simulink model "sim_aut_dual_scen"  (R2025b)
settings: Solver=ode45  StartTime=0.0  StopTime=Tfin  FixedStep=1e-3  MaxStep=1e-2  MinStep=1e-3  RelTol=5e-3
values from neighbouring files (symbols this model uses):
  bp = [-1.25 -1.19897959184 -1.14795918367 -1.09693877551 -1.04591836735 -0.994897959184 -0.94387755102 -0.892857142857 -0.841836734694 -0.790816326531 -0.739795918367 -0.688775510204 ... (50 elements, 1x50)]    [tire_model.mat]
  C1 = 2.7e4    (= 27000)    [main.m]    (also in model.m)
  C2 = 2e4    (= 20000)    [main.m]    (also in model.m)
  Jz = 4000    [main.m]    (also in model.m)
  K = nmpc_design_st2(par,2)    [main.m]
  l1 = 1.2    [main.m]    (also in model.m)
  l2 = 1.6    [main.m]    (also in model.m)
  m = 1575    [main.m]    (also in model.m)
  Np = round(vx_ref*K.Tp/mean(ds))    [main.m]
  pacf = [2550.90487699 2674.70463742 2810.77279096 2960.97362657 3127.55760929 3313.26346728 3521.4532226 3756.29269015 4022.99538347 4328.15571957 4680.20907939 5090.07319782 ... (50 elements, 1x50)]    [tire_model.mat]
  pacr = [2550.90487699 2674.70463742 2810.77279096 2960.97362657 3127.55760929 3313.26346728 3521.4532226 3756.29269015 4022.99538347 4328.15571957 4680.20907939 5090.07319782 ... (50 elements, 1x50)]    [tire_model.mat]
  psi = x(3)    [model.m]
  psir = [atan2(diff(Yr),diff(Xr));0]    [main.m]
  refPoses = [Xr,Yr,psir]    [main.m]
  Ts = 0.05    [main.m]
  ze0 = [X0;Y0;psi0;vx0;vy0;wpsi0]    [main.m]
undefined symbols (not defined in the file or in its folder): aMode, plot_ref, x_o
libraries: autolibsharedcommon x11, autolibshared x5, autolibpowerinfoutils x2, autolibutils x2, sharedtransform x2, simulink x1, drivingscenarioandsensors x1
(part 2 of 4)

== system sim_aut_dual_scen/vehicle/dual-track/Vehicle Body 3DOF Dual Track/friction/mu ext dual ==
  mu_in : Inport  PortDimensions=[2,2]
  Signal Specification1 : SignalSpecification  Unit=1
  Unit Conversion2 : UnitConversion
  mu_out : Outport  PortDimensions=[2,2]  VectorParamsAs1DForOutWhenUnconnected=off
  wires:
  Signal Specification1/1 -> mu_out/1
  mu_in/1 -> Unit Conversion2/1
  Unit Conversion2/1 -> Signal Specification1/1

== system sim_aut_dual_scen/vehicle/dual-track/Vehicle Body 3DOF Dual Track/friction/mu int ==
  Constant : Constant  Value=mu
  Vector Concatenate1 : Concatenate
  mu_out : Outport  VectorParamsAs1DForOutWhenUnconnected=off
  wires:
  Constant/1 -> Vector Concatenate1/1, Vector Concatenate1/2
  Vector Concatenate1/1 -> mu_out/1

== system sim_aut_dual_scen/vehicle/dual-track/Vehicle Body 3DOF Dual Track/friction/mu int dual ==
  Constant : Constant  Value=mu
  Vector Concatenate2 : Concatenate  Mode=Multidimensional array  ConcatenateDimension=2
  Vector Concatenate3 : Concatenate  Mode=Multidimensional array  ConcatenateDimension=2
  Vector Concatenate4 : Concatenate  Mode=Multidimensional array
  mu_out : Outport  VectorParamsAs1DForOutWhenUnconnected=off
  wires:
  Vector Concatenate2/1 -> Vector Concatenate4/1
  Vector Concatenate3/1 -> Vector Concatenate4/2
  Vector Concatenate4/1 -> mu_out/1
  Constant/1 -> Vector Concatenate3/2, Vector Concatenate3/1, Vector Concatenate2/2, Vector Concatenate2/1

== system sim_aut_dual_scen/vehicle/dual-track/Vehicle Body 3DOF Dual Track/front forces/ext ==
  F_in : Inport  PortDimensions=2
  Signal Specification1 : SignalSpecification  Unit=N
  Unit Conversion3 : UnitConversion
  F_out : Outport  Unit=N  VectorParamsAs1DForOutWhenUnconnected=off
  wires:
  Signal Specification1/1 -> F_out/1
  F_in/1 -> Unit Conversion3/1
  Unit Conversion3/1 -> Signal Specification1/1

== system sim_aut_dual_scen/vehicle/dual-track/Vehicle Body 3DOF Dual Track/front forces/ext dual ==
  F_in : Inport  PortDimensions=[2,2]
  Signal Specification1 : SignalSpecification  Unit=N
  Unit Conversion3 : UnitConversion
  F_out : Outport  Unit=N  PortDimensions=[2,2]  VectorParamsAs1DForOutWhenUnconnected=off
  wires:
  Signal Specification1/1 -> F_out/1
  F_in/1 -> Unit Conversion3/1
  Unit Conversion3/1 -> Signal Specification1/1

== system sim_aut_dual_scen/vehicle/dual-track/Vehicle Body 3DOF Dual Track/front forces/ext long ==
  F_in : Inport
  Ground1 : Ground
  Signal Specification : SignalSpecification  Unit=N
  Signal Specification1 : SignalSpecification  Unit=N
  Unit Conversion1 : UnitConversion
  Vector Concatenate1 : Concatenate
  F_out : Outport  Unit=N  VectorParamsAs1DForOutWhenUnconnected=off
  wires:
  Signal Specification/1 -> Vector Concatenate1/2
  F_in/1 -> Unit Conversion1/1
  Vector Concatenate1/1 -> F_out/1
  Ground1/1 -> Signal Specification/1
  Unit Conversion1/1 -> Signal Specification1/1
  Signal Specification1/1 -> Vector Concatenate1/1

== system sim_aut_dual_scen/vehicle/dual-track/Vehicle Body 3DOF Dual Track/front forces/ext long dual ==
  F_in : Inport
  Demux : Demux  Outputs=2
  Ground : Ground
  Signal Specification5 : SignalSpecification  Unit=N
  Unit Conversion2 : UnitConversion  OutputType=Inherit: Inherit via back propagation
  Vector Concatenate1 : Concatenate  Mode=Multidimensional array  ConcatenateDimension=2
  Vector Concatenate2 : Concatenate  Mode=Multidimensional array  ConcatenateDimension=2
  Vector Concatenate3 : Concatenate  Mode=Multidimensional array
  F_out : Outport  Unit=N  VectorParamsAs1DForOutWhenUnconnected=off
  wires:
  Ground/1 -> Vector Concatenate2/2, Vector Concatenate1/2
  Vector Concatenate3/1 -> F_out/1
  Vector Concatenate1/1 -> Vector Concatenate3/1
  Vector Concatenate2/1 -> Vector Concatenate3/2
  Demux/1 -> Vector Concatenate1/1
  Demux/2 -> Vector Concatenate2/1
  Unit Conversion2/1 -> Signal Specification5/1
  Signal Specification5/1 -> Demux/1
  F_in/1 -> Unit Conversion2/1

== system sim_aut_dual_scen/vehicle/dual-track/Vehicle Body 3DOF Dual Track/front forces/int ==
  Ground : Ground
  Vector Concatenate1 : Concatenate
  F_out : Outport  VectorParamsAs1DForOutWhenUnconnected=off
  wires:
  Ground/1 -> Vector Concatenate1/2, Vector Concatenate1/1
  Vector Concatenate1/1 -> F_out/1

== system sim_aut_dual_scen/vehicle/dual-track/Vehicle Body 3DOF Dual Track/front forces/int dual ==
  Ground : Ground
  Vector Concatenate2 : Concatenate  Mode=Multidimensional array  ConcatenateDimension=2
  Vector Concatenate3 : Concatenate  Mode=Multidimensional array  ConcatenateDimension=2
  Vector Concatenate4 : Concatenate  Mode=Multidimensional array
  F_out : Outport  VectorParamsAs1DForOutWhenUnconnected=off
  wires:
  Vector Concatenate2/1 -> Vector Concatenate4/1
  Vector Concatenate3/1 -> Vector Concatenate4/2
  Vector Concatenate4/1 -> F_out/1
  Ground/1 -> Vector Concatenate3/2, Vector Concatenate3/1, Vector Concatenate2/2, Vector Concatenate2/1

== system sim_aut_dual_scen/vehicle/dual-track/Vehicle Body 3DOF Dual Track/front steer/delta ext ==
  delta_in : Inport  Unit=rad
  Signal Specification1 : SignalSpecification  Unit=rad
  Unit Conversion1 : UnitConversion
  delta_out : Outport  VectorParamsAs1DForOutWhenUnconnected=off
  wires:
  Signal Specification1/1 -> delta_out/1
  Unit Conversion1/1 -> Signal Specification1/1
  delta_in/1 -> Unit Conversion1/1

== system sim_aut_dual_scen/vehicle/dual-track/Vehicle Body 3DOF Dual Track/front steer/delta ext dual ==
  delta_in : Inport  PortDimensions=2
  Signal Specification1 : SignalSpecification  Unit=rad
  Unit Conversion2 : UnitConversion
  delta_out : Outport  Unit=rad  PortDimensions=2  VectorParamsAs1DForOutWhenUnconnected=off
  wires:
  Signal Specification1/1 -> delta_out/1
  Unit Conversion2/1 -> Signal Specification1/1
  delta_in/1 -> Unit Conversion2/1

== system sim_aut_dual_scen/vehicle/dual-track/Vehicle Body 3DOF Dual Track/front steer/delta int ==
  Ground : Ground
  delta_out : Outport  VectorParamsAs1DForOutWhenUnconnected=off
  wires:
  Ground/1 -> delta_out/1

== system sim_aut_dual_scen/vehicle/dual-track/Vehicle Body 3DOF Dual Track/front steer/delta int dual ==
  Constant : Constant  Value=0
  Vector Concatenate4 : Concatenate
  delta_out : Outport  VectorParamsAs1DForOutWhenUnconnected=off
  wires:
  Constant/1 -> Vector Concatenate4/1, Vector Concatenate4/2
  Vector Concatenate4/1 -> delta_out/1

== system sim_aut_dual_scen/vehicle/dual-track/Vehicle Body 3DOF Dual Track/hitch geometry parameters/hitch active bicycle ==
  Constant : Constant  Value=dh
  Constant1 : Constant  Value=hh
  Ground : Ground
  dh_out : Outport  VectorParamsAs1DForOutWhenUnconnected=off
  hh_out : Outport  Port=2  VectorParamsAs1DForOutWhenUnconnected=off
  hl_out : Outport  Port=3  VectorParamsAs1DForOutWhenUnconnected=off
  wires:
  Ground/1 -> hl_out/1
  Constant1/1 -> hh_out/1
  Constant/1 -> dh_out/1

== system sim_aut_dual_scen/vehicle/dual-track/Vehicle Body 3DOF Dual Track/hitch geometry parameters/hitch active dual track ==
  Constant : Constant  Value=dh
  Constant1 : Constant  Value=hh
  Constant2 : Constant  Value=hl
  dh_out : Outport  VectorParamsAs1DForOutWhenUnconnected=off
  hh_out : Outport  Port=2  VectorParamsAs1DForOutWhenUnconnected=off
  hl_out : Outport  Port=3  VectorParamsAs1DForOutWhenUnconnected=off
  wires:
  Constant2/1 -> hl_out/1
  Constant1/1 -> hh_out/1
  Constant/1 -> dh_out/1

== system sim_aut_dual_scen/vehicle/dual-track/Vehicle Body 3DOF Dual Track/hitch geometry parameters/hitch inactive ==
  Ground : Ground
  dh_out : Outport  Unit=m  PortDimensions=1  VectorParamsAs1DForOutWhenUnconnected=off
  hh_out : Outport  Port=2  Unit=m  PortDimensions=1  VectorParamsAs1DForOutWhenUnconnected=off
  hl_out : Outport  Port=3  Unit=m  PortDimensions=1  VectorParamsAs1DForOutWhenUnconnected=off
  wires:
  Ground/1 -> dh_out/1, hh_out/1, hl_out/1

== system sim_aut_dual_scen/vehicle/dual-track/Vehicle Body 3DOF Dual Track/sigma/no sigma ==
  y : Inport
  Demux : Demux  Outputs=2
  Selector : Selector  InputPortWidth=4  IndexOptions=Index vector (dialog)  Indices=[1,3]  OutputSizes=1
  alpha_f : Outport  VectorParamsAs1DForOutWhenUnconnected=off
  alpha_r : Outport  Port=2  VectorParamsAs1DForOutWhenUnconnected=off
  wires:
  Demux/2 -> alpha_r/1
  Demux/1 -> alpha_f/1
  Selector/1 -> Demux/1
  y/1 -> Selector/1

== system sim_aut_dual_scen/vehicle/dual-track/Vehicle Body 3DOF Dual Track/sigma/no sigma dual ==
  y : Inport  PortDimensions=8
  Demux : Demux  Outputs=[2,2,4]
  Terminator : Terminator
  alpha_f : Outport  VectorParamsAs1DForOutWhenUnconnected=off
  alpha_r : Outport  Port=2  VectorParamsAs1DForOutWhenUnconnected=off
  wires:
  y/1 -> Demux/1
  Demux/1 -> alpha_f/1
  Demux/2 -> alpha_r/1
  Demux/3 -> Terminator/1

== system sim_aut_dual_scen/vehicle/dual-track/Vehicle Body 3DOF Dual Track/sigma/sigma ==
  y : Inport
  Constant1 : Constant  Value=sigma_f
  Constant2 : Constant  Value=sigma_r
  Demux : Demux
  relaxation front : Subsystem
  relaxation rear : Subsystem
  alpha_f : Outport  VectorParamsAs1DForOutWhenUnconnected=off
  alpha_r : Outport  Port=2  VectorParamsAs1DForOutWhenUnconnected=off
  wires:
  Demux/3 -> relaxation rear/1(alpha)
  y/1 -> Demux/1
  Constant1/1 -> relaxation front/3(sigma)
  Constant2/1 -> relaxation rear/3(sigma)
  Demux/2 -> relaxation front/2(V)
  Demux/4 -> relaxation rear/2(V)
  relaxation rear/1(alpha_sig) -> alpha_r/1
  Demux/1 -> relaxation front/1(alpha)
  relaxation front/1(alpha_sig) -> alpha_f/1

== system sim_aut_dual_scen/vehicle/dual-track/Vehicle Body 3DOF Dual Track/sigma/sigma dual ==
  y : Inport  PortDimensions=8
  Constant1 : Constant  Value=sigma_f
  Constant2 : Constant  Value=sigma_r
  Demux : Demux  Outputs=[4,4]
  Demux1 : Demux  Outputs=[2,2]
  Vector Concatenate : Concatenate  NumInputs=4
  relaxation : Subsystem
  alpha_f : Outport  VectorParamsAs1DForOutWhenUnconnected=off
  alpha_r : Outport  Port=2  VectorParamsAs1DForOutWhenUnconnected=off
  wires:
  relaxation/1(alpha_sig) -> Demux1/1
  Demux/1 -> relaxation/1(alpha)
  Demux/2 -> relaxation/2(V)
  y/1 -> Demux/1
  Constant1/1 -> Vector Concatenate/2, Vector Concatenate/1
  Constant2/1 -> Vector Concatenate/3, Vector Concatenate/4
  Vector Concatenate/1 -> relaxation/3(sigma)
  Demux1/1 -> alpha_f/1
  Demux1/2 -> alpha_r/1

== system sim_aut_dual_scen/vehicle/dual-track/Vehicle Body 3DOF Dual Track/sigma1/no sigma ==
  y : Inport
  Demux : Demux  Outputs=2
  Selector : Selector  InputPortWidth=4  IndexOptions=Index vector (dialog)  Indices=[1,3]  OutputSizes=1
  alpha_f : Outport  VectorParamsAs1DForOutWhenUnconnected=off
  alpha_r : Outport  Port=2  VectorParamsAs1DForOutWhenUnconnected=off
  wires:
  y/1 -> Selector/1
  Selector/1 -> Demux/1
  Demux/1 -> alpha_f/1
  Demux/2 -> alpha_r/1

== system sim_aut_dual_scen/vehicle/dual-track/Vehicle Body 3DOF Dual Track/sigma1/no sigma dual ==
  y : Inport  PortDimensions=8
  Demux : Demux  Outputs=[2,2,4]
  Terminator : Terminator
  alpha_f : Outport  VectorParamsAs1DForOutWhenUnconnected=off
  alpha_r : Outport  Port=2  VectorParamsAs1DForOutWhenUnconnected=off
  wires:
  Demux/3 -> Terminator/1
  Demux/2 -> alpha_r/1
  Demux/1 -> alpha_f/1
  y/1 -> Demux/1

== system sim_aut_dual_scen/vehicle/dual-track/Vehicle Body 3DOF Dual Track/sigma1/sigma ==
  y : Inport
  Constant1 : Constant  Value=sigma_f
  Constant2 : Constant  Value=sigma_r
  Demux : Demux
  relaxation front : Subsystem
  relaxation rear : Subsystem
  alpha_f : Outport  VectorParamsAs1DForOutWhenUnconnected=off
  alpha_r : Outport  Port=2  VectorParamsAs1DForOutWhenUnconnected=off
  wires:
  relaxation front/1(alpha_sig) -> alpha_f/1
  Demux/1 -> relaxation front/1(alpha)
  relaxation rear/1(alpha_sig) -> alpha_r/1
  Demux/4 -> relaxation rear/2(V)
  Demux/2 -> relaxation front/2(V)
  Constant2/1 -> relaxation rear/3(sigma)
  Constant1/1 -> relaxation front/3(sigma)
  y/1 -> Demux/1
  Demux/3 -> relaxation rear/1(alpha)

== system sim_aut_dual_scen/vehicle/dual-track/Vehicle Body 3DOF Dual Track/sigma1/sigma dual ==
  y : Inport  PortDimensions=8
  Demux : Demux  Outputs=[4,4]
  Demux1 : Demux  Outputs=[2,2]
  Terminator : Terminator
  relaxation : Subsystem
  alpha_f : Outport  VectorParamsAs1DForOutWhenUnconnected=off
  alpha_r : Outport  Port=2  VectorParamsAs1DForOutWhenUnconnected=off
  wires:
  Demux1/2 -> alpha_r/1
  Demux1/1 -> alpha_f/1
  y/1 -> Demux/1
  Demux/1 -> relaxation/1(alpha)
  relaxation/1(alpha_sig) -> Demux1/1
  Demux/2 -> Terminator/1

== system sim_aut_dual_scen/vehicle/dual-track/Vehicle Body 3DOF Dual Track/state/xdot ext ==
  xdot : Inport
  xddot_in : Inport  Port=2  PortDimensions=4
  extState : Inport  Port=3
  Integrator : Integrator  InitialConditionSource=external  InitialCondition=[x_o;ydot_o;psi;r_o;x_o;xdot_o]
  Selector : Selector  InputPortWidth=4  IndexOptions=Index vector (dialog)  Indices=[2:4]  OutputSizes=1
  Selector1 : Selector  InputPortWidth=4  IndexOptions=Index vector (dialog)  Indices=[2:4]  OutputSizes=1
  Signal Specification : SignalSpecification  Unit=m/s
  Unit Conversion6 : UnitConversion
  Vector Concatenate : Concatenate
  Vector Concatenate1 : Concatenate
  xddot_out : Outport  VectorParamsAs1DForOutWhenUnconnected=off
  wires:
  Selector1/1 -> Vector Concatenate/2
  extState/1 -> Selector1/1
  xddot_in/1 -> Integrator/1
  Vector Concatenate1/1 -> xddot_out/1
  Selector/1 -> Vector Concatenate1/2
  xdot/1 -> Unit Conversion6/1
  Vector Concatenate/1 -> Integrator/2
  Integrator/1 -> Selector/1
  Unit Conversion6/1 -> Signal Specification/1
  Signal Specification/1 -> Vector Concatenate/1, Vector Concatenate1/1

== system sim_aut_dual_scen/vehicle/dual-track/Vehicle Body 3DOF Dual Track/state/xdot int ==
  xddot_in : Inport  PortDimensions=4
  extState : Inport  Port=2
  Integrator : Integrator  InitialConditionSource=external  InitialCondition=[x_o;ydot_o;psi;r_o;x_o;xdot_o]
  xddot_out : Outport  VectorParamsAs1DForOutWhenUnconnected=off
  wires:
  extState/1 -> Integrator/2
  xddot_in/1 -> Integrator/1
  Integrator/1 -> xddot_out/1

== system sim_aut_dual_scen/vehicle/dual-track/Vehicle Body 3DOF Dual Track/wind/wind ext ==
  wind_in : Inport
  Signal Specification1 : SignalSpecification  Unit=m/s
  Unit Conversion5 : UnitConversion
  wind_out : Outport  Unit=m/s  VectorParamsAs1DForOutWhenUnconnected=off
  wires:
  Signal Specification1/1 -> wind_out/1
  wind_in/1 -> Unit Conversion5/1
  Unit Conversion5/1 -> Signal Specification1/1

== system sim_aut_dual_scen/vehicle/dual-track/Vehicle Body 3DOF Dual Track/wind/wind int ==
  Ground : Ground
  Vector Concatenate1 : Concatenate  NumInputs=3
  wind_out : Outport  Unit=m/s  VectorParamsAs1DForOutWhenUnconnected=off
  wires:
  Ground/1 -> Vector Concatenate1/1, Vector Concatenate1/2, Vector Concatenate1/3
  Vector Concatenate1/1 -> wind_out/1

== system sim_aut_dual_scen/vehicle/dual-track/Vehicle Body 3DOF Dual Track/Cy/Cy table dual/For Each Subsystem ==
  alpha_f : Inport  Partition=on  PartitionDimension=1  PartitionWidth=1  PartitionOffset=0
  alpha_r : Inport  Port=2  Partition=on  PartitionDimension=1  PartitionWidth=1  PartitionOffset=0
  Cy_f(alpha_f) : Lookup_n-D  NumberOfTableDimensions=1  BreakpointsForDimension1=alpha_f_brk  Table=Cy_f_data  ExtrapMethod=Clip  InternalRulePriority=Speed  RndMeth=Simplest
  Cy_r(alpha_r) : Lookup_n-D  NumberOfTableDimensions=1  BreakpointsForDimension1=alpha_r_brk  Table=Cy_r_data  ExtrapMethod=Clip  InternalRulePriority=Speed  RndMeth=Simplest
  For Each : ForEach  DisableCoverage=on
  Cy_f : Outport  ConcatenationDimension=1  VectorParamsAs1DForOutWhenUnconnected=off
  Cy_r : Outport  Port=2  ConcatenationDimension=1  VectorParamsAs1DForOutWhenUnconnected=off
  wires:
  Cy_r(alpha_r)/1 -> Cy_r/1
  alpha_r/1 -> Cy_r(alpha_r)/1
  Cy_f(alpha_f)/1 -> Cy_f/1
  alpha_f/1 -> Cy_f(alpha_f)/1

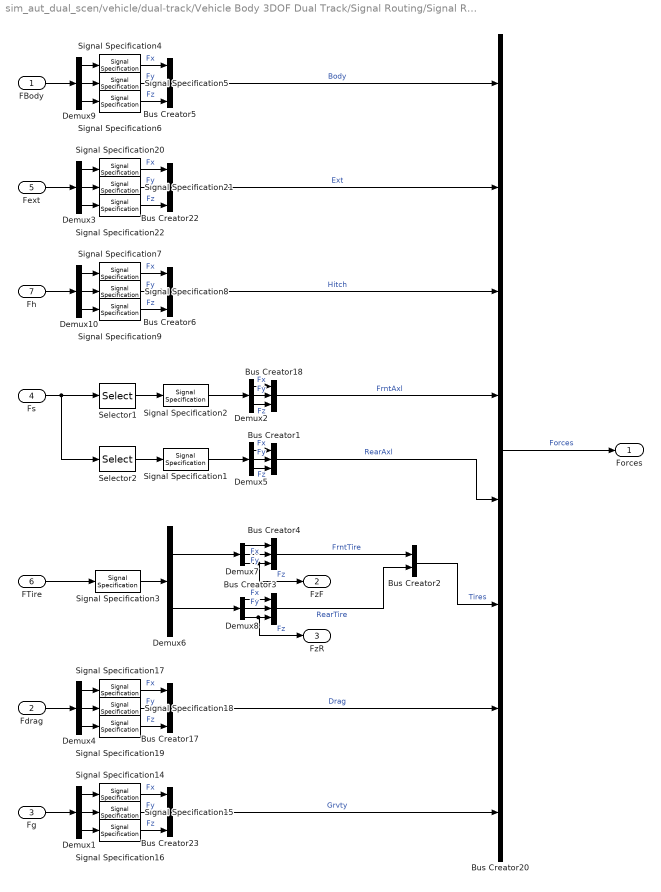
== system sim_aut_dual_scen/vehicle/dual-track/Vehicle Body 3DOF Dual Track/Signal Routing/Signal Routing/Forces 3DOF ==
  FBody : Inport
  Fdrag : Inport  Port=2
  Fg : Inport  Port=3
  Fs : Inport  Port=4  Unit=N
  Fext : Inport  Port=5
  FTire : Inport  Port=6
  Fh : Inport  Port=7  Unit=N
  Bus Creator{1,3..6,17..18,22..23} (9 alike) : BusCreator  Inputs=3
  Bus Creator2 : BusCreator  Inputs=2
  Bus Creator20 : BusCreator  Inputs=8
  Demux{1..5,7..10} (9 alike) : Demux  Outputs=3
  Demux6 : Demux  Outputs=[3,3]
  Selector1 : Selector  IndexOptions=Index vector (dialog)  Indices=[1:3]  OutputSizes=1
  Selector2 : Selector  IndexOptions=Index vector (dialog)  Indices=[4:6]  OutputSizes=1
  Signal Specification{1..9,14..22} (18 alike) : SignalSpecification  Unit=N
  Forces : Outport  VectorParamsAs1DForOutWhenUnconnected=off
  FzF : Outport  Port=2  VectorParamsAs1DForOutWhenUnconnected=off
  FzR : Outport  Port=3  VectorParamsAs1DForOutWhenUnconnected=off
  wires:
  Signal Specification8/1 -> Bus Creator6/2  "Fy"
  Fh/1 -> Demux10/1
  Signal Specification7/1 -> Bus Creator6/1  "Fx"
  Demux10/3 -> Signal Specification9/1
  Demux10/1 -> Signal Specification7/1
  Bus Creator6/1 -> Bus Creator20/3  "Hitch"
  Signal Specification9/1 -> Bus Creator6/3  "Fz"
  Demux10/2 -> Signal Specification8/1
  Signal Specification5/1 -> Bus Creator5/2  "Fy"
  Signal Specification4/1 -> Bus Creator5/1  "Fx"
  Signal Specification6/1 -> Bus Creator5/3  "Fz"
  FBody/1 -> Demux9/1
  Demux9/1 -> Signal Specification4/1
  Demux9/2 -> Signal Specification5/1
  Demux9/3 -> Signal Specification6/1
  Bus Creator5/1 -> Bus Creator20/1  "Body"
  Bus Creator17/1 -> Bus Creator20/7  "Drag"
  Bus Creator2/1 -> Bus Creator20/6  "Tires"
  Demux6/2 -> Demux8/1
  Demux6/1 -> Demux7/1
  Signal Specification3/1 -> Demux6/1
  FTire/1 -> Signal Specification3/1
  Selector2/1 -> Signal Specification1/1
  Signal Specification2/1 -> Demux2/1
  Signal Specification1/1 -> Demux5/1
  Fs/1 -> Selector2/1, Selector1/1
  Selector1/1 -> Signal Specification2/1
  Demux5/1 -> Bus Creator1/1  "Fx"
  Bus Creator4/1 -> Bus Creator2/1  "FrntTire"
  Bus Creator3/1 -> Bus Creator2/2  "RearTire"
  Demux7/1 -> Bus Creator4/1  "Fx"
  Demux7/2 -> Bus Creator4/2  "Fy"
  Demux7/3 -> Bus Creator4/3, FzF/1  "Fz"
  Demux8/3 -> Bus Creator3/3, FzR/1  "Fz"
  Demux8/2 -> Bus Creator3/2  "Fy"
  Demux8/1 -> Bus Creator3/1  "Fx"
  Demux5/2 -> Bus Creator1/2  "Fy"
  Demux5/3 -> Bus Creator1/3  "Fz"
  Demux2/3 -> Bus Creator18/3  "Fz"
  Demux2/2 -> Bus Creator18/2  "Fy"
  Demux2/1 -> Bus Creator18/1  "Fx"
  Bus Creator1/1 -> Bus Creator20/5  "RearAxl"
  Bus Creator18/1 -> Bus Creator20/4  "FrntAxl"
  Fdrag/1 -> Demux4/1
  Demux4/3 -> Signal Specification19/1
  Demux4/2 -> Signal Specification18/1
  Demux4/1 -> Signal Specification17/1
  Demux3/3 -> Signal Specification22/1
  Demux3/2 -> Signal Specification21/1
  Demux3/1 -> Signal Specification20/1
  Fext/1 -> Demux3/1
  Bus Creator22/1 -> Bus Creator20/2  "Ext"
  Signal Specification22/1 -> Bus Creator22/3  "Fz"
  Signal Specification20/1 -> Bus Creator22/1  "Fx"
  Signal Specification15/1 -> Bus Creator23/2  "Fy"
  Signal Specification21/1 -> Bus Creator22/2  "Fy"
  Signal Specification18/1 -> Bus Creator17/2  "Fy"
  Signal Specification17/1 -> Bus Creator17/1  "Fx"
  Signal Specification14/1 -> Bus Creator23/1  "Fx"
  Signal Specification19/1 -> Bus Creator17/3  "Fz"
  Signal Specification16/1 -> Bus Creator23/3  "Fz"
  Bus Creator20/1 -> Forces/1  "Forces"
  Bus Creator23/1 -> Bus Creator20/8  "Grvty"
  Demux1/2 -> Signal Specification15/1
  Demux1/3 -> Signal Specification16/1
  Fg/1 -> Demux1/1
  Demux1/1 -> Signal Specification14/1

== system sim_aut_dual_scen/vehicle/dual-track/Vehicle Body 3DOF Dual Track/Signal Routing/Signal Routing/Lateral 3DOF ==
  InertCg : Inport
  BdyFrmCg : Inport  Port=2
  Forces : Inport  Port=3
  Power : Inport  Port=4
  Moments : Inport  Port=5
  WhlAngF : Inport  Port=6  Unit=rad
  WhlAngR : Inport  Port=7  Unit=rad
  Bus Creator1 : BusCreator  Inputs=8
  Bus Creator2 : BusCreator  Inputs=5
  Bus Creator3 : BusCreator  Inputs=2
  Bus Creator4 : BusCreator  Inputs=2
  Bus Selector : BusSelector  OutputSignals=Pwr,PwrInfo
  Demux : Demux  Outputs=2
  Demux1 : Demux  Outputs=2
  Hard Point Coordinate Transform Front : autolibsharedcommon/Hard Point Coordinate Transform  R_T1=a  R_T2=0  R_T3=h  aMode=aMode
  Hard Point Coordinate Transform Geometric : Subsystem
  Hard Point Coordinate Transform Rear : autolibsharedcommon/Hard Point Coordinate Transform  R_T1=-b  R_T2=0  R_T3=h  aMode=aMode
  Hitch Coordinate Transform : Subsystem
  InertFrm : Outport  VectorParamsAs1DForOutWhenUnconnected=off
  BdyFrm : Outport  Port=2  VectorParamsAs1DForOutWhenUnconnected=off
  PwrInfo : Outport  Port=3  VectorParamsAs1DForOutWhenUnconnected=off
  wires:
  Hitch Coordinate Transform/1(Inert) -> Bus Creator2/4  "Hitch"
  Hitch Coordinate Transform/2(Body) -> Bus Creator1/6  "Hitch"
  Bus Creator2/1 -> InertFrm/1
  InertCg/1 -> Hard Point Coordinate Transform Geometric/1(InertFrmCg), Hitch Coordinate Transform/1(InertFrmCg), Hard Point Coordinate Transform Rear/1, Hard Point Coordinate Transform Front/1, Bus Creator2/1  "Cg"
  Hard Point Coordinate Transform Front/1 -> Bus Creator2/2  "FrntAxl"
  Hard Point Coordinate Transform Rear/2 -> Bus Creator1/5  "RearAxl"
  Bus Creator1/1 -> BdyFrm/1  "BdyFrm"
  Hard Point Coordinate Transform Rear/1 -> Bus Creator2/3  "RearAxl"
  Hard Point Coordinate Transform Front/2 -> Bus Creator1/4  "FrntAxl"
  Forces/1 -> Bus Creator1/2  "Forces"
  Bus Selector/1 -> Bus Creator1/7  "<Pwr>"
  Moments/1 -> Bus Creator1/3  "Moments"
  BdyFrmCg/1 -> Hard Point Coordinate Transform Front/2, Hitch Coordinate Transform/2(BodyFrmCg), Bus Creator1/1, Hard Point Coordinate Transform Geometric/2(BdyFrmCg), Hard Point Coordinate Transform Rear/2  "Cg"
  Hard Point Coordinate Transform Geometric/1(Inert) -> Bus Creator2/5  "Geom"
  Hard Point Coordinate Transform Geometric/2(Body) -> Bus Creator1/8  "Geom"
  Bus Creator3/1 -> Hard Point Coordinate Transform Front/3  "Steer"
  WhlAngF/1 -> Demux/1  "WhlAngF"
  WhlAngR/1 -> Demux1/1  "WhlAngR"
  Bus Creator4/1 -> Hard Point Coordinate Transform Rear/3  "Steer"
  Demux/2 -> Bus Creator3/2  "WhlAngFR"
  Demux1/1 -> Bus Creator4/1  "WhlAngRL"
  Demux1/2 -> Bus Creator4/2  "WhlAngRR"
  Demux/1 -> Bus Creator3/1  "WhlAngFL"
  Bus Selector/2 -> PwrInfo/1  "<PwrInfo>"
  Power/1 -> Bus Selector/1  "Pwr"

== system sim_aut_dual_scen/vehicle/dual-track/Vehicle Body 3DOF Dual Track/Signal Routing/Signal Routing/Moments ==
  MBody : Inport
  Mdrag : Inport  Port=2
  MExt : Inport  Port=3
  Mh : Inport  Port=4
  Bus Creator{1..3,24} (4 alike) : BusCreator  Inputs=3
  Bus Creator7 : BusCreator  Inputs=4
  Demux{,1..3} (4 alike) : Demux  Outputs=3
  Signal Specification{1..11,23} (12 alike) : SignalSpecification  Unit=N*m
  Moments : Outport  VectorParamsAs1DForOutWhenUnconnected=off
  wires:
  Signal Specification10/1 -> Bus Creator2/3  "Mz"
  Demux3/3 -> Signal Specification10/1
  Demux3/1 -> Signal Specification11/1
  Signal Specification11/1 -> Bus Creator2/1  "Mx"
  Mh/1 -> Demux3/1
  Demux3/2 -> Signal Specification9/1
  Signal Specification9/1 -> Bus Creator2/2  "My"
  Bus Creator2/1 -> Bus Creator7/4  "Hitch"
  Signal Specification23/1 -> Bus Creator24/1  "Mx"
  Bus Creator24/1 -> Bus Creator7/1  "Body"
  Signal Specification1/1 -> Bus Creator24/2  "My"
  Signal Specification2/1 -> Bus Creator24/3  "Mz"
  Bus Creator1/1 -> Bus Creator7/2  "Drag"
  Bus Creator7/1 -> Moments/1  "Moments"
  Demux/2 -> Signal Specification1/1
  Demux/1 -> Signal Specification23/1
  Demux/3 -> Signal Specification2/1
  MBody/1 -> Demux/1
  Mdrag/1 -> Demux1/1
  Demux1/3 -> Signal Specification4/1
  Demux1/1 -> Signal Specification5/1
  Demux1/2 -> Signal Specification3/1
  Signal Specification4/1 -> Bus Creator1/3  "Mz"
  Signal Specification3/1 -> Bus Creator1/2  "My"
  Signal Specification5/1 -> Bus Creator1/1  "Mx"
  MExt/1 -> Demux2/1
  Signal Specification7/1 -> Bus Creator3/3  "Mz"
  Signal Specification6/1 -> Bus Creator3/2  "My"
  Bus Creator3/1 -> Bus Creator7/3  "Ext"
  Signal Specification8/1 -> Bus Creator3/1  "Mx"
  Demux2/2 -> Signal Specification6/1
  Demux2/1 -> Signal Specification8/1
  Demux2/3 -> Signal Specification7/1

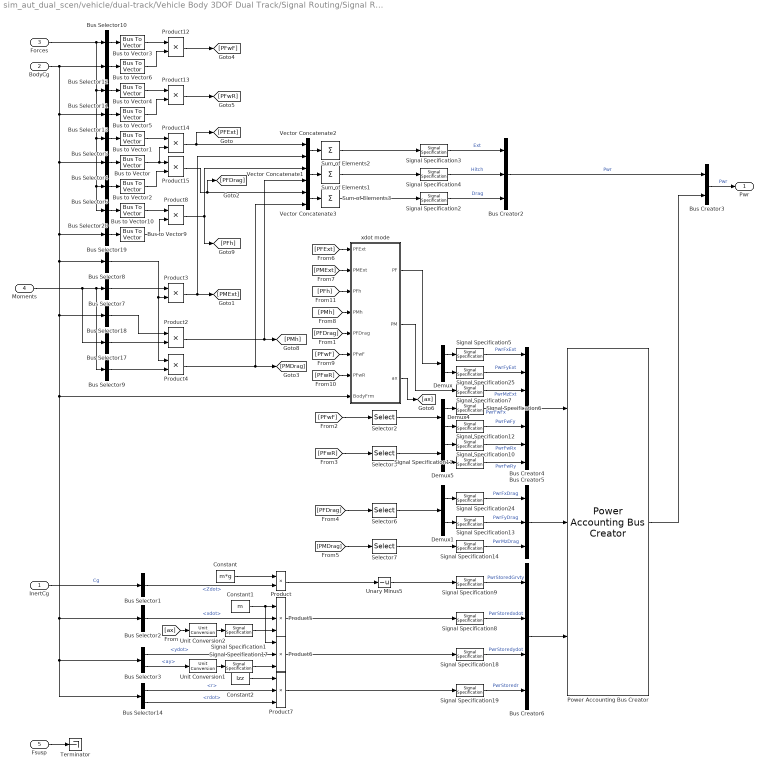
== system sim_aut_dual_scen/vehicle/dual-track/Vehicle Body 3DOF Dual Track/Signal Routing/Signal Routing/Power ==
  InertCg : Inport
  BodyCg : Inport  Port=2
  Forces : Inport  Port=3
  Moments : Inport  Port=4
  Fsusp : Inport  Port=5
  Bus Creator2 : BusCreator  Inputs=3
  Bus Creator3 : BusCreator  Inputs=2
  Bus Creator4 : BusCreator  Inputs=7
  Bus Creator5 : BusCreator  Inputs=3
  Bus Creator6 : BusCreator  Inputs=4
  Bus Selector1 : BusSelector  OutputSignals=Cg.Vel.Zdot
  Bus Selector10 : BusSelector  OutputSignals=FrntAxl.Fx,FrntAxl.Fy,FrntAxl.Fz  OutputAsBus=on
  Bus Selector11 : BusSelector  OutputSignals=RearAxl.Fx,RearAxl.Fy,RearAxl.Fz  OutputAsBus=on
  Bus Selector12 : BusSelector  OutputSignals=FrntAxl.Vel.xdot,FrntAxl.Vel.ydot,FrntAxl.Vel.zdot  OutputAsBus=on
  Bus Selector13 : BusSelector  OutputSignals=RearAxl.Vel.xdot,RearAxl.Vel.ydot,RearAxl.Vel.zdot  OutputAsBus=on
  Bus Selector14 : BusSelector  OutputSignals=Cg.AngVel.r,Cg.AngAcc.rdot
  Bus Selector17 : BusSelector  OutputSignals=Hitch.Mx,Hitch.My,Hitch.Mz  OutputAsBus=on
  Bus Selector18 : BusSelector  OutputSignals=Cg.AngVel.p,Cg.AngVel.q,Cg.AngVel.r  OutputAsBus=on
  Bus Selector19 : BusSelector  OutputSignals=Hitch.Vel.xdot,Hitch.Vel.ydot,Hitch.Vel.zdot  OutputAsBus=on
  Bus Selector2 : BusSelector  OutputSignals=Cg.Vel.xdot
  Bus Selector20 : BusSelector  OutputSignals=Hitch.Fx,Hitch.Fy,Hitch.Fz  OutputAsBus=on
  Bus Selector3 : BusSelector  OutputSignals=Cg.Vel.ydot,Cg.Acc.ay
  Bus Selector4 : BusSelector  OutputSignals=Cg.Vel.xdot,Cg.Vel.ydot,Cg.Vel.zdot  OutputAsBus=on
  Bus Selector5 : BusSelector  OutputSignals=Ext.Fx,Ext.Fy,Ext.Fz  OutputAsBus=on
  Bus Selector6 : BusSelector  OutputSignals=Drag.Fx,Drag.Fy,Drag.Fz  OutputAsBus=on
  Bus Selector7 : BusSelector  OutputSignals=Ext.Mx,Ext.My,Ext.Mz  OutputAsBus=on
  Bus Selector8 : BusSelector  OutputSignals=Cg.AngVel.p,Cg.AngVel.q,Cg.AngVel.r  OutputAsBus=on
  Bus Selector9 : BusSelector  OutputSignals=Drag.Mx,Drag.My,Drag.Mz  OutputAsBus=on
  Bus to Vector{,1..6,9..10} (9 alike) : BusToVector
  Constant : Constant  Value=m*g
  Constant1 : Constant  Value=m
  Constant2 : Constant  Value=Izz
  Demux{,1,4..5} (4 alike) : Demux  Outputs=2
  Power Accounting Bus Creator : autolibpowerinfoutils/Power Accounting Bus Creator  AssctBlkSelPopup=Parent reference block  RefBlkName='autolibshared/Vehicle Body 3DOF Single Track'  PwrTrnsfrdCheckBox=on  PwrNotTrnsfrdCheckBox=on  PwrStoredCheckBox=on  aMode=aMode
  Product{,2..4,8,12..15} (9 alike) : Product
  Product5 : Product  Inputs=3
  Product6 : Product  Inputs=3
  Product7 : Product  Inputs=3
  Selector2 : Selector  InputPortWidth=3  IndexOptions=Index vector (dialog)  Indices=[1 2]  OutputSizes=1
  Selector3 : Selector  InputPortWidth=3  IndexOptions=Index vector (dialog)  Indices=[1 2]  OutputSizes=1
  Selector6 : Selector  InputPortWidth=3  IndexOptions=Index vector (dialog)  Indices=[1 2]  OutputSizes=1
  Selector7 : Selector  InputPortWidth=3  IndexOptions=Index vector (dialog)  Indices=[3]  OutputSizes=1
  Signal Specification1 : SignalSpecification  Unit=m/s^2
  Signal Specification{2..14,18..19,24..25} (17 alike) : SignalSpecification  Unit=W
  Signal Specification17 : SignalSpecification  Unit=m/s^2
  Sum of Elements1 : Sum  Inputs=+
  Sum of Elements2 : Sum  Inputs=+
  Sum of Elements3 : Sum  Inputs=+
  Terminator : Terminator
  Unary Minus5 : UnaryMinus
  Unit Conversion1 : UnitConversion
  Unit Conversion2 : UnitConversion
  Vector Concatenate1 : Concatenate
  Vector Concatenate2 : Concatenate
  Vector Concatenate3 : Concatenate
  xdot mode : Subsystem  Variant=on  VariantControlMode=label  LabelModeActiveChoice=1
  Pwr : Outport  VectorParamsAs1DForOutWhenUnconnected=off
  wires:
  [PMh] -> xdot mode/4(PMh)
  [PFh] -> xdot mode/3(PFh)
  Vector Concatenate1/1 -> Sum of Elements1/1
  Sum of Elements1/1 -> Signal Specification4/1
  Signal Specification4/1 -> Bus Creator2/2  "Hitch"
  Bus Selector19/1 -> Bus to Vector9/1
  Bus to Vector9/1 -> Product8/2
  Bus to Vector10/1 -> Product8/1
  Bus Selector20/1 -> Bus to Vector10/1
  Product8/1 -> [PFh], Vector Concatenate1/1
  Product2/1 -> Vector Concatenate1/2, [PMh]
  BodyCg/1 -> Bus Selector4/1, Bus Selector8/1, Bus Selector18/1, xdot mode/8(BodyFrm), Bus Selector2/1, Bus Selector14/1, Bus Selector3/1, Bus Selector19/1, Bus Selector13/1, Bus Selector12/1
  Moments/1 -> Bus Selector7/1, Bus Selector9/1, Bus Selector17/1
  Bus Selector18/1 -> Product2/1
  Bus Selector17/1 -> Product2/2
  Signal Specification3/1 -> Bus Creator2/1  "Ext"
  Product15/1 -> Vector Concatenate3/1, [PFDrag]
  Bus Creator2/1 -> Bus Creator3/1  "Pwr"
  Product14/1 -> [PFExt], Vector Concatenate2/1
  Bus Selector5/1 -> Bus to Vector1/1
  Bus Selector1/1 -> Product/2  "<Zdot>"
  Product3/1 -> [PMExt], Vector Concatenate2/2
  Bus Selector11/1 -> Bus to Vector4/1
  InertCg/1 -> Bus Selector1/1  "Cg"
  Sum of Elements3/1 -> Signal Specification2/1
  Bus to Vector1/1 -> Product14/1
  Bus Selector6/1 -> Bus to Vector2/1
  Signal Specification8/1 -> Bus Creator6/2  "PwrStoredxdot"
  [PFwR] -> Selector3/1
  Demux/2 -> Signal Specification25/1
  Product13/1 -> [PFwR]
  Product7/1 -> Signal Specification19/1
  Bus Selector3/1 -> Product6/2  "<ydot>"
  Constant2/1 -> Product7/1
  Sum of Elements2/1 -> Signal Specification3/1
  Bus to Vector2/1 -> Product15/2
  Bus Selector13/1 -> Bus to Vector5/1
  Vector Concatenate2/1 -> Sum of Elements2/1
  Signal Specification19/1 -> Bus Creator6/4  "PwrStoredr"
  Bus Selector2/1 -> Product5/2  "<xdot>"
  Vector Concatenate3/1 -> Sum of Elements3/1
  Signal Specification18/1 -> Bus Creator6/3  "PwrStoredydot"
  Bus Selector14/2 -> Product7/3  "<rdot>"
  Bus Selector14/1 -> Product7/2  "<r>"
  Forces/1 -> Bus Selector6/1, Bus Selector20/1, Bus Selector5/1, Bus Selector11/1, Bus Selector10/1
  xdot mode/1(PF) -> Demux/1
  Bus Selector10/1 -> Bus to Vector3/1
  Bus to Vector6/1 -> Product12/2
  [PMDrag] -> Selector7/1
  Signal Specification14/1 -> Bus Creator5/3  "PwrMzDrag"
  [PFwF] -> Selector2/1
  Signal Specification7/1 -> Bus Creator4/3  "PwrMzExt"
  Bus Selector4/1 -> Bus to Vector/1
  Bus to Vector3/1 -> Product12/1
  Signal Specification13/1 -> Bus Creator5/2  "PwrFyDrag"
  [PFDrag] -> Selector6/1
  Selector6/1 -> Demux1/1
  Bus Selector12/1 -> Bus to Vector6/1
  Signal Specification6/1 -> Bus Creator4/4  "PwrFwFx"
  Bus Creator3/1 -> Pwr/1  "Pwr"
  Bus to Vector4/1 -> Product13/1
  Signal Specification9/1 -> Bus Creator6/1  "PwrStoredGrvty"
  Signal Specification11/1 -> Bus Creator4/7  "PwrFwRy"
  xdot mode/2(PM) -> Signal Specification7/1
  Bus Selector7/1 -> Product3/1
  Signal Specification2/1 -> Bus Creator2/3  "Drag"
  Bus Selector8/1 -> Product3/2, Product4/1
  Signal Specification10/1 -> Bus Creator4/6  "PwrFwRx"
  Signal Specification12/1 -> Bus Creator4/5  "PwrFwFy"
  Selector2/1 -> Demux4/1
  Demux5/2 -> Signal Specification11/1
  Bus Selector9/1 -> Product4/2
  Selector3/1 -> Demux5/1
  Demux4/1 -> Signal Specification6/1
  Demux1/1 -> Signal Specification24/1
  Product12/1 -> [PFwF]
  Unary Minus5/1 -> Signal Specification9/1
  Signal Specification24/1 -> Bus Creator5/1  "PwrFxDrag"
  Demux5/1 -> Signal Specification10/1
  Signal Specification5/1 -> Bus Creator4/1  "PwrFxExt"
  Bus Creator6/1 -> Power Accounting Bus Creator/3
  Bus to Vector/1 -> Product15/1, Product14/2
  Constant1/1 -> Product6/1, Product5/1
  Signal Specification25/1 -> Bus Creator4/2  "PwrFyExt"
  Product/1 -> Unary Minus5/1
  Bus Creator5/1 -> Power Accounting Bus Creator/2
  Bus to Vector5/1 -> Product13/2
  Bus Creator4/1 -> Power Accounting Bus Creator/1
  Demux/1 -> Signal Specification5/1
  Product6/1 -> Signal Specification18/1
  Constant/1 -> Product/1
  Demux4/2 -> Signal Specification12/1
  Power Accounting Bus Creator/1 -> Bus Creator3/2
  Product4/1 -> [PMDrag], Vector Concatenate3/2
  Fsusp/1 -> Terminator/1
  [PFExt] -> xdot mode/1(PFExt)
  [PMExt] -> xdot mode/2(PMExt)
  [PFDrag] -> xdot mode/5(PFDrag)
  [PFwF] -> xdot mode/6(PFwF)
  [PFwR] -> xdot mode/7(PFwR)
  Product5/1 -> Signal Specification8/1
  Signal Specification17/1 -> Product6/3
  Unit Conversion1/1 -> Signal Specification17/1
  Bus Selector3/2 -> Unit Conversion1/1  "<ay>"
  Selector7/1 -> Signal Specification14/1
  Demux1/2 -> Signal Specification13/1
  Signal Specification1/1 -> Product5/3
  Unit Conversion2/1 -> Signal Specification1/1
  xdot mode/3(ax) -> [ax]
  [ax] -> Unit Conversion2/1

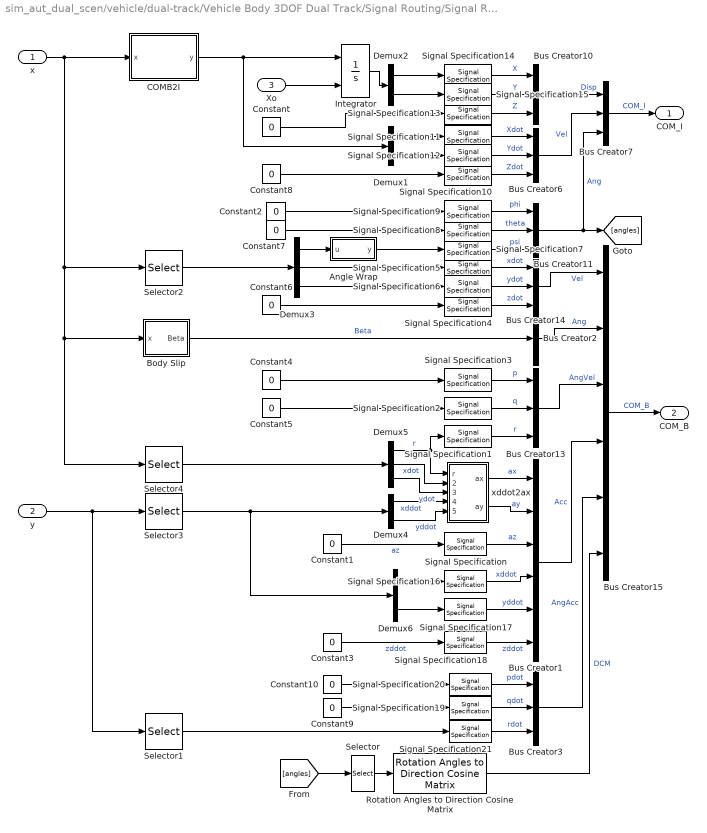
== system sim_aut_dual_scen/vehicle/dual-track/Vehicle Body 3DOF Dual Track/Signal Routing/Signal Routing/state2bus ==
  x : Inport
  y : Inport  Port=2
  Xo : Inport  Port=3
  Angle Wrap : Subsystem  Variant=on  VariantControlMode=label  VariantControl=Variant1  LabelModeActiveChoice=None
  Body Slip : Subsystem
  Bus Creator1 : BusCreator  Inputs=6
  Bus Creator{3,6..7,10..11,13..14} (7 alike) : BusCreator  Inputs=3
  Bus Creator15 : BusCreator  Inputs=6
  Bus Creator2 : BusCreator  Inputs=1
  COMB2I : MATLAB Function  TreatAsAtomicUnit=on
  Constant{,1..10} (11 alike) : Constant  Value=0
  Demux{1..2,4,6} (4 alike) : Demux  Outputs=2
  Demux3 : Demux  Outputs=3
  Demux5 : Demux  Outputs=3
  Integrator : Integrator  InitialConditionSource=external
  Rotation Angles to Direction Cosine Matrix : sharedtransform/Rotation Angles to Direction Cosine Matrix  rotationOrder=ZYX  aMode=aMode
  Selector : Selector  InputPortWidth=3  IndexOptions=Index vector (dialog)  Indices=[3 2 1]  OutputSizes=1
  Selector1 : Selector  IndexOptions=Index vector (dialog)  Indices=[3]  OutputSizes=1
  Selector2 : Selector  IndexOptions=Index vector (dialog)  Indices=[3,1,2]  OutputSizes=1
  Selector3 : Selector  IndexOptions=Index vector (dialog)  Indices=[1,2]  OutputSizes=1
  Selector4 : Selector  IndexOptions=Index vector (dialog)  Indices=[4,1,2]  OutputSizes=1
  Signal Specification : SignalSpecification  Unit=gn
  Signal Specification1 : SignalSpecification  Unit=rad/s
  Signal Specification{4..6,10..12} (6 alike) : SignalSpecification  Unit=m/s
  Signal Specification13 : SignalSpecification  Unit=m
  Signal Specification14 : SignalSpecification  Unit=m
  Signal Specification15 : SignalSpecification  Unit=m
  Signal Specification16 : SignalSpecification  Unit=m/s^2
  Signal Specification17 : SignalSpecification  Unit=m/s^2
  Signal Specification18 : SignalSpecification  Unit=m/s^2
  Signal Specification19 : SignalSpecification  Unit=rad/s^2
  Signal Specification2 : SignalSpecification  Unit=rad/s
  Signal Specification20 : SignalSpecification  Unit=rad/s^2
  Signal Specification21 : SignalSpecification  Unit=rad/s^2
  Signal Specification3 : SignalSpecification  Unit=rad/s
  Signal Specification7 : SignalSpecification  Unit=rad
  Signal Specification8 : SignalSpecification  Unit=rad
  Signal Specification9 : SignalSpecification  Unit=rad
  xddot2ax : Subsystem
  COM_I : Outport  VectorParamsAs1DForOutWhenUnconnected=off
  COM_B : Outport  Port=2  VectorParamsAs1DForOutWhenUnconnected=off
  wires:
  [angles] -> Selector/1
  Selector/1 -> Rotation Angles to Direction Cosine Matrix/1
  Rotation Angles to Direction Cosine Matrix/1 -> Bus Creator15/6  "DCM"
  Angle Wrap/1(" y") -> Signal Specification7/1
  Selector1/1 -> Signal Specification21/1
  Constant10/1 -> Signal Specification20/1
  Constant9/1 -> Signal Specification19/1
  Bus Creator3/1 -> Bus Creator15/5  "AngAcc"
  Signal Specification20/1 -> Bus Creator3/1  "pdot"
  Signal Specification19/1 -> Bus Creator3/2  "qdot"
  Signal Specification21/1 -> Bus Creator3/3  "rdot"
  Xo/1 -> Integrator/2
  Body Slip/1(Beta) -> Bus Creator2/1  "Beta"
  Bus Creator2/1 -> Bus Creator15/2  "Ang"
  Bus Creator1/1 -> Bus Creator15/4  "Acc"
  Constant8/1 -> Signal Specification10/1
  Demux6/2 -> Signal Specification17/1
  Demux6/1 -> Signal Specification16/1
  Constant1/1 -> Signal Specification/1  "az"
  Signal Specification16/1 -> Bus Creator1/4  "xddot"
  Signal Specification17/1 -> Bus Creator1/5  "yddot"
  Signal Specification18/1 -> Bus Creator1/6  "zddot"
  Constant3/1 -> Signal Specification18/1  "zddot"
  Selector3/1 -> Demux6/1, Demux4/1
  y/1 -> Selector3/1, Selector1/1
  Signal Specification/1 -> Bus Creator1/3  "az"
  Signal Specification7/1 -> Bus Creator11/3  "psi"
  COMB2I/1(y) -> Demux1/1, Integrator/1
  Integrator/1 -> Demux2/1
  Signal Specification6/1 -> Bus Creator14/2  "ydot"
  Bus Creator11/1 -> Bus Creator7/3, [angles]  "Ang"
  Signal Specification5/1 -> Bus Creator14/1  "xdot"
  Bus Creator15/1 -> COM_B/1  "COM_B"
  Signal Specification2/1 -> Bus Creator13/2  "q"
  Signal Specification12/1 -> Bus Creator6/2  "Ydot"
  Selector2/1 -> Demux3/1
  Signal Specification8/1 -> Bus Creator11/2  "theta"
  Bus Creator10/1 -> Bus Creator7/1  "Disp"
  Bus Creator6/1 -> Bus Creator7/2  "Vel"
  Bus Creator14/1 -> Bus Creator15/1  "Vel"
  Signal Specification3/1 -> Bus Creator13/1  "p"
  Bus Creator7/1 -> COM_I/1  "COM_I"
  Signal Specification9/1 -> Bus Creator11/1  "phi"
  Signal Specification14/1 -> Bus Creator10/1  "X"
  Signal Specification13/1 -> Bus Creator10/3  "Z"
  Bus Creator13/1 -> Bus Creator15/3  "AngVel"
  Signal Specification15/1 -> Bus Creator10/2  "Y"
  Signal Specification11/1 -> Bus Creator6/1  "Xdot"
  Signal Specification4/1 -> Bus Creator14/3  "zdot"
  Signal Specification10/1 -> Bus Creator6/3  "Zdot"
  x/1 -> COMB2I/1(x), Selector2/1, Body Slip/1(x), Selector4/1
  Demux5/1 -> Signal Specification1/1, xddot2ax/1(r)  "r"
  Selector4/1 -> Demux5/1
  Demux5/2 -> xddot2ax/2(xdot)  "xdot"
  Demux5/3 -> xddot2ax/3(ydot)  "ydot"
  Demux4/1 -> xddot2ax/4(xddot)  "xddot"
  Demux4/2 -> xddot2ax/5(yddot)  "yddot"
  xddot2ax/1(ax) -> Bus Creator1/1  "ax"
  xddot2ax/2(ay) -> Bus Creator1/2  "ay"
  Signal Specification1/1 -> Bus Creator13/3  "r"
  Constant5/1 -> Signal Specification2/1
  Constant4/1 -> Signal Specification3/1
  Constant6/1 -> Signal Specification4/1
  Demux3/2 -> Signal Specification5/1
  Demux3/3 -> Signal Specification6/1
  Demux3/1 -> Angle Wrap/1("u ")
  Constant7/1 -> Signal Specification8/1
  Constant2/1 -> Signal Specification9/1
  Demux1/2 -> Signal Specification12/1
  Demux1/1 -> Signal Specification11/1
  Constant/1 -> Signal Specification13/1
  Demux2/2 -> Signal Specification15/1
  Demux2/1 -> Signal Specification14/1

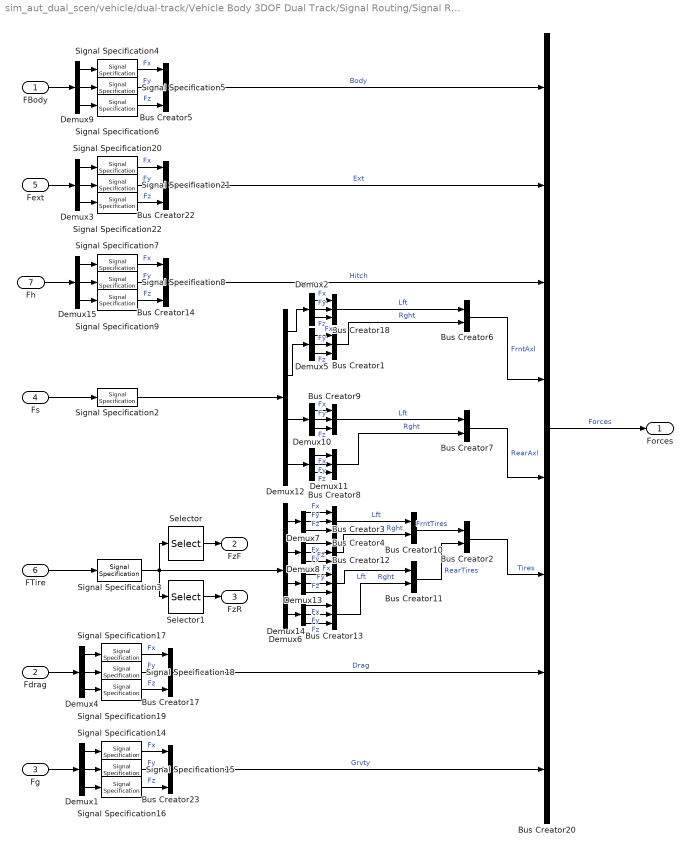
== system sim_aut_dual_scen/vehicle/dual-track/Vehicle Body 3DOF Dual Track/Signal Routing/Signal Routing Dual/Forces 3DOF ==
  FBody : Inport
  Fdrag : Inport  Port=2
  Fg : Inport  Port=3
  Fs : Inport  Port=4  Unit=N
  Fext : Inport  Port=5
  FTire : Inport  Port=6
  Fh : Inport  Port=7
  Bus Creator{1,3..5,8..9,12..14,17..18,22..23} (13 alike) : BusCreator  Inputs=3
  Bus Creator{2,6..7,10..11} (5 alike) : BusCreator  Inputs=2
  Bus Creator20 : BusCreator  Inputs=8
  Demux{1..5,7..11,13..15} (13 alike) : Demux  Outputs=3
  Demux12 : Demux  Outputs=[3,3,3,3]
  Demux6 : Demux  Outputs=[3,3,3,3]
  Selector : Selector  InputPortWidth=12  IndexOptions=Index vector (dialog)  Indices=[3,6]  OutputSizes=1
  Selector1 : Selector  InputPortWidth=12  IndexOptions=Index vector (dialog)  Indices=[9,12]  OutputSizes=1
  Signal Specification{2..9,14..22} (17 alike) : SignalSpecification  Unit=N
  Forces : Outport  VectorParamsAs1DForOutWhenUnconnected=off
  FzF : Outport  Port=2  VectorParamsAs1DForOutWhenUnconnected=off
  FzR : Outport  Port=3  VectorParamsAs1DForOutWhenUnconnected=off
  wires:
  Demux15/2 -> Signal Specification8/1
  Demux15/1 -> Signal Specification7/1
  Signal Specification9/1 -> Bus Creator14/3  "Fz"
  Signal Specification8/1 -> Bus Creator14/2  "Fy"
  Fh/1 -> Demux15/1
  Demux15/3 -> Signal Specification9/1
  Bus Creator14/1 -> Bus Creator20/3  "Hitch"
  Signal Specification7/1 -> Bus Creator14/1  "Fx"
  Selector1/1 -> FzR/1
  Selector/1 -> FzF/1
  Demux13/3 -> Bus Creator12/3  "Fz"
  Bus Creator13/1 -> Bus Creator11/2  "Rght"
  Demux14/1 -> Bus Creator13/1  "Fx"
  Demux14/2 -> Bus Creator13/2  "Fy"
  Demux14/3 -> Bus Creator13/3  "Fz"
  Demux6/4 -> Demux14/1
  Demux6/3 -> Demux13/1
  Demux13/2 -> Bus Creator12/2  "Fy"
  Demux13/1 -> Bus Creator12/1  "Fx"
  Signal Specification2/1 -> Demux12/1
  Bus Creator12/1 -> Bus Creator11/1  "Lft"
  Bus Creator3/1 -> Bus Creator10/2  "Rght"
  Bus Creator4/1 -> Bus Creator10/1  "Lft"
  Demux12/3 -> Demux10/1
  Demux12/4 -> Demux11/1
  Demux11/1 -> Bus Creator8/1  "Fx"
  Demux11/2 -> Bus Creator8/2  "Fy"
  Demux11/3 -> Bus Creator8/3  "Fz"
  Demux10/3 -> Bus Creator9/3  "Fz"
  Demux10/2 -> Bus Creator9/2  "Fy"
  Demux10/1 -> Bus Creator9/1  "Fx"
  Bus Creator9/1 -> Bus Creator7/1  "Lft"
  Bus Creator8/1 -> Bus Creator7/2  "Rght"
  Bus Creator1/1 -> Bus Creator6/2  "Rght"
  Bus Creator18/1 -> Bus Creator6/1  "Lft"
  Demux1/1 -> Signal Specification14/1
  Fg/1 -> Demux1/1
  Demux1/3 -> Signal Specification16/1
  Demux1/2 -> Signal Specification15/1
  Bus Creator23/1 -> Bus Creator20/8  "Grvty"
  Bus Creator20/1 -> Forces/1  "Forces"
  Signal Specification16/1 -> Bus Creator23/3  "Fz"
  Signal Specification19/1 -> Bus Creator17/3  "Fz"
  Signal Specification14/1 -> Bus Creator23/1  "Fx"
  Signal Specification17/1 -> Bus Creator17/1  "Fx"
  Signal Specification18/1 -> Bus Creator17/2  "Fy"
  Signal Specification21/1 -> Bus Creator22/2  "Fy"
  Signal Specification15/1 -> Bus Creator23/2  "Fy"
  Signal Specification20/1 -> Bus Creator22/1  "Fx"
  Signal Specification22/1 -> Bus Creator22/3  "Fz"
  Bus Creator22/1 -> Bus Creator20/2  "Ext"
  Fext/1 -> Demux3/1
  Demux3/1 -> Signal Specification20/1
  Demux3/2 -> Signal Specification21/1
  Demux3/3 -> Signal Specification22/1
  Demux4/1 -> Signal Specification17/1
  Demux4/2 -> Signal Specification18/1
  Demux4/3 -> Signal Specification19/1
  Fdrag/1 -> Demux4/1
  Bus Creator6/1 -> Bus Creator20/4  "FrntAxl"
  Bus Creator7/1 -> Bus Creator20/5  "RearAxl"
  Demux2/1 -> Bus Creator18/1  "Fx"
  Demux2/2 -> Bus Creator18/2  "Fy"
  Demux2/3 -> Bus Creator18/3  "Fz"
  Demux5/3 -> Bus Creator1/3  "Fz"
  Demux5/2 -> Bus Creator1/2  "Fy"
  Demux8/1 -> Bus Creator3/1  "Fx"
  Demux8/2 -> Bus Creator3/2  "Fy"
  Demux8/3 -> Bus Creator3/3  "Fz"
  Demux7/3 -> Bus Creator4/3  "Fz"
  Demux7/2 -> Bus Creator4/2  "Fy"
  Demux7/1 -> Bus Creator4/1  "Fx"
  Bus Creator11/1 -> Bus Creator2/2  "RearTires"
  Bus Creator10/1 -> Bus Creator2/1  "FrntTires"
  Demux5/1 -> Bus Creator1/1  "Fx"
  Fs/1 -> Signal Specification2/1
  Demux12/2 -> Demux5/1
  Demux12/1 -> Demux2/1
  FTire/1 -> Signal Specification3/1
  Signal Specification3/1 -> Demux6/1, Selector/1, Selector1/1
  Demux6/1 -> Demux7/1
  Demux6/2 -> Demux8/1
  Bus Creator2/1 -> Bus Creator20/6  "Tires"
  Bus Creator17/1 -> Bus Creator20/7  "Drag"
  Bus Creator5/1 -> Bus Creator20/1  "Body"
  Demux9/3 -> Signal Specification6/1
  Demux9/2 -> Signal Specification5/1
  Demux9/1 -> Signal Specification4/1
  FBody/1 -> Demux9/1
  Signal Specification6/1 -> Bus Creator5/3  "Fz"
  Signal Specification4/1 -> Bus Creator5/1  "Fx"
  Signal Specification5/1 -> Bus Creator5/2  "Fy"

== system sim_aut_dual_scen/vehicle/dual-track/Vehicle Body 3DOF Dual Track/Signal Routing/Signal Routing Dual/Lateral 3DOF ==
  InertCg : Inport
  BdyFrmCg : Inport  Port=2
  Forces : Inport  Port=3
  Power : Inport  Port=4
  Moments : Inport  Port=5
  WhlAngF : Inport  Port=6
  WhlAngR : Inport  Port=7
  Bus Creator1 : BusCreator  Inputs=8
  Bus Creator2 : BusCreator  Inputs=5
  Bus Creator{3..4,7..8} (4 alike) : BusCreator  Inputs=2
  Bus Creator5 : BusCreator  Inputs=3
  Bus Creator6 : BusCreator  Inputs=3
  Bus Selector : BusSelector  OutputSignals=Pwr,PwrInfo
  Demux : Demux  Outputs=2
  Demux1 : Demux  Outputs=2
  Hard Point Coordinate Transform Front Left : Subsystem
  Hard Point Coordinate Transform Front Right : Subsystem
  Hard Point Coordinate Transform Geometric : Subsystem
  Hard Point Coordinate Transform Rear Left : Subsystem
  Hard Point Coordinate Transform Rear Right : Subsystem
  Hitch Coordinate Transform : Subsystem
  InertFrm : Outport  VectorParamsAs1DForOutWhenUnconnected=off
  BdyFrm : Outport  Port=2  VectorParamsAs1DForOutWhenUnconnected=off
  PwrInfo : Outport  Port=3  VectorParamsAs1DForOutWhenUnconnected=off
  wires:
  Hitch Coordinate Transform/2(Body) -> Bus Creator1/6  "Hitch"
  Hitch Coordinate Transform/1(Inert) -> Bus Creator2/4  "Hitch"
  Power/1 -> Bus Selector/1  "Pwr"
  Bus Selector/1 -> Bus Creator1/7  "<Pwr>"
  Bus Selector/2 -> PwrInfo/1  "<PwrInfo>"
  Demux1/2 -> Bus Creator7/2  "WhlAngRR"
  Demux1/1 -> Bus Creator7/1  "WhlAngRL"
  Demux/2 -> Bus Creator8/2  "WhlAngFR"
  Demux/1 -> Bus Creator8/1  "WhlAngFL"
  Bus Creator8/1 -> Bus Creator5/3  "Steer"
  Bus Creator7/1 -> Bus Creator6/3  "Steer"
  WhlAngR/1 -> Demux1/1  "WhlAngR"
  WhlAngF/1 -> Demux/1  "WhlAngF"
  Hard Point Coordinate Transform Geometric/1(Inert) -> Bus Creator2/5  "Geom"
  Hard Point Coordinate Transform Geometric/2(Body) -> Bus Creator1/8  "Geom"
  Forces/1 -> Bus Creator1/2  "Forces"
  BdyFrmCg/1 -> Hard Point Coordinate Transform Front Left/2(BdyFrmCg), Hard Point Coordinate Transform Front Right/2(BdyFrmCg), Hard Point Coordinate Transform Rear Left/2(BdyFrmCg), Hard Point Coordinate Transform Rear Right/2(BdyFrmCg), Hitch Coordinate Transform/2(BodyFrmCg), Bus Creator1/1, Hard Point Coordinate Transform Geometric/2(BdyFrmCg)  "Cg"
  Bus Creator3/1 -> Bus Creator2/2  "FrntAxl"
  Bus Creator1/1 -> BdyFrm/1  "BdyFrm"
  Bus Creator2/1 -> InertFrm/1  "InertFrm"
  Bus Creator4/1 -> Bus Creator2/3  "RearAxl"
  InertCg/1 -> Hard Point Coordinate Transform Rear Left/1(InertFrmCg), Hard Point Coordinate Transform Rear Right/1(InertFrmCg), Hard Point Coordinate Transform Geometric/1(InertFrmCg), Hitch Coordinate Transform/1(InertFrmCg), Hard Point Coordinate Transform Front Right/1(InertFrmCg), Bus Creator2/1, Hard Point Coordinate Transform Front Left/1(InertFrmCg)  "Cg"
  Bus Creator5/1 -> Bus Creator1/4  "FrntAxl"
  Moments/1 -> Bus Creator1/3  "Moments"
  Hard Point Coordinate Transform Front Left/1(Inert) -> Bus Creator3/1  "Lft"
  Hard Point Coordinate Transform Front Right/1(Inert) -> Bus Creator3/2  "Rght"
  Hard Point Coordinate Transform Rear Left/1(Inert) -> Bus Creator4/1  "Lft"
  Hard Point Coordinate Transform Rear Right/1(Inert) -> Bus Creator4/2  "Rght"
  Hard Point Coordinate Transform Rear Right/2(Body) -> Bus Creator6/2  "Rght"
  Hard Point Coordinate Transform Rear Left/2(Body) -> Bus Creator6/1  "Lft"
  Hard Point Coordinate Transform Front Right/2(Body) -> Bus Creator5/2  "Rght"
  Hard Point Coordinate Transform Front Left/2(Body) -> Bus Creator5/1  "Lft"
  Bus Creator6/1 -> Bus Creator1/5  "RearAxl"
